simulink model "s5"  (Simulink 2.00)
settings: Solver=ode15s  StartTime=0.0  StopTime=tstop  MaxStep=1e-2  RelTol=1e-6  AbsTol=1e-6
values from neighbouring files (symbols this model uses):
  Domega = 0    [I3ESSR.M]    (also in M3.M; M3G.M; M5.M = 1; SET1.M = 2)
  H = 2.89    [I3ESSR.M]    (also in M1.M = 0.5*J_rotor*wbasem*wbasem/Sbase; M3.M = diag(h); M3G.M = diag(h); M5.M = 0.352825293175)
  IdeIqe = polyfit(Iqe',Ide',2)    [M5.M]
  Ipm = Em/xmd    [M5.M]
  Psido = xls*(-Ido) + Psiado    [M1.M]    (also in M3.M = xls*(-Ido) + Psimdo; M3G.M = xls*(-Ido) + Psimdo; M5.M = Psiado)
  Psiqo = xls*(-Iqo) + Psiaqo    [M1.M]    (also in M3.M = xls*(-Iqo) + Psimqo; M3G.M = xls*(-Iqo) + Psimqo; M5.M = 0)
  rs = 0.00    (= 0)    [I3ESSR.M]    (also in M1.M = rs/Zbase; M3.M; M3G.M = 0.001; M5.M = rs/Zb)
  VsTem = polyfit(Tem',Vs',2)    [M5.M]
  wb = wbase    [M1.M]    (also in M2.M = 376.991118431; M3.M = 376.991118431; M3G.M = 376.991118431; M4.M = we)
  wrbywbo = 0    [M5.M]
  xd = 1.79    [I3ESSR.M]    (also in M1.M = xd/Zbase; M3.M; M3G.M; M5.M = xd/Zb)
  xls = 0.13    [I3ESSR.M]    (also in M1.M = xls/Zbase; M3.M; M3G.M; M5.M = xls/Zb)
  xmd = xmd/Zbase    [M1.M]    (also in M3.M = 1.66; M3G.M = 1.66; M5.M = xmd/Zb)
  xMD = (1/xls + 1/xmd + 1/xplf + 1/xplkd)^(-1)    [M1.M]    (also in M3.M = 0.00484867453082; M3G.M = 0.00484867453082; M5.M = 0.0152325462012)
  xMQ = (1/xls + 1/xmq + 1/xplkq)^(-1)    [M1.M]    (also in M3.M = 0.0456224786115; M3G.M = 0.0456224786115; M5.M = 0.0170549070248)
  xq = 1.71    [I3ESSR.M]    (also in M1.M = xq/Zbase; M3.M; M3G.M; M5.M = xq/Zb)
  Zb = Vb/Ib    [M5.M]
settings Model: SaveTime=off  SaveOutput=off  ConsistencyChecking=off

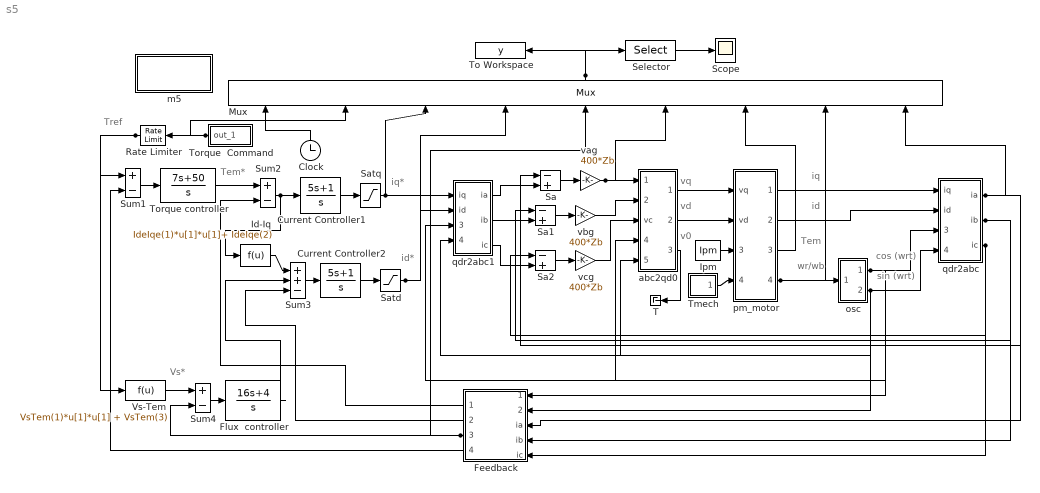
== system s5 ==
  note: Tem
  note: wr/wb
  note: cos (wrt)
  note: sin (wrt)
  note: id
  note: iq
  note: Vs*
  note: Tem*
  note: Tref
  note: id*
  note: iq*
  note: vq
  note: vd
  note: v0
  Clock : Clock
      settings: Orientation=up  DeleteFcn=simclock BlockIsBeingDestroyed  PostSaveFcn=simclock Save
  Current Controller1 : TransferFcn  Numerator=[5 1]  Denominator=[1 0]
  Current Controller2 : TransferFcn  Numerator=[5 1]  Denominator=[1 0]
  Feedback : Subsystem  Orientation=left
  Flux  controller : TransferFcn  Numerator=[16 4]  Denominator=[1 0]
  Id-Iq : Fcn  Expr=IdeIqe(1)*u[1]*u[1]+ IdeIqe(2)
  Ipm : Constant  Value=Ipm
  m5 : Subsystem
      settings: OpenFcn=m5
      mask Type: Masked block of m5.m
      mask Help: Uses m5.m to initialize and plot
      mask Display: disp('Initialize\nand plot')
  Mux : Mux  Orientation=up  Inputs=9
  Rate Limiter : RateLimiter  Orientation=left  RisingSlewLimit=1000  FallingSlewLimit=-1000
  Sa : Sum  Inputs=-+
  Sa1 : Sum  Inputs=-+
  Sa2 : Sum  Inputs=-+
  Satd : Saturate  UpperLimit=1.2  LowerLimit=-1.2
  Satq : Saturate  UpperLimit=1.2  LowerLimit=-1.2
  Scope : Scope
      settings: TickLabels=on  TimeRange=3  YMin=-1  YMax=1  SaveToWorkspace=off  SaveName=ScopeData  LimitMaxRows=off
  Selector : Selector  Elements=[2 5 6 7 8 9]  InputPortWidth=9
  Sum1 : Sum  Inputs=+-
  Sum2 : Sum  Inputs=+-
  Sum3 : Sum  Inputs=++-
  Sum4 : Sum  Inputs=+-
  T : Terminator
  Tmech : Subsystem  mask(Repeating table){@1=tmech_time, @2=tmech_value}
      mask prompts: @1 "Time values:"; @2 "Output values:"
      mask help:
      | Repeating table.
      | Enter values of time and output for first cycle.
      mask init:
      | period = max(@1); t = @1; y = @2;
      mask Help: Repeats cycle given in table. Time values should be monotonically increasing.
      mask Display: plot([t,t+period,t+2*period],[y,y,y])
  To Workspace : ToWorkspace  VariableName=y  SampleTime=0
      settings: Buffer=40000
  Torque controller : TransferFcn  Numerator=[7 50]  Denominator=[1 0]
  Torque  Command : Subsystem  Orientation=left  mask(Repeating table){@1=tref_time, @2=tref_value}
      mask prompts: @1 "Time values:"; @2 "Output values:"
      mask help:
      | Repeating table.
      | Enter values of time and output for first cycle.
      mask init:
      | period = max(@1); t = @1; y = @2;
      mask Help: Repeats cycle given in table. Time values should be monotonically increasing.
      mask Display: plot([t,t+period,t+2*period],[y,y,y])
  Vs-Tem : Fcn  Expr=VsTem(1)*u[1]*u[1] + VsTem(3)
  abc2qd0 : Subsystem
  osc : Subsystem
  pm_motor : Subsystem
  qdr2abc : Subsystem
  qdr2abc1 : Subsystem
  vag : Gain  Gain=400*Zb
  vbg : Gain  Gain=400*Zb
  vcg : Gain  Gain=400*Zb
  wires:
  Mux/1 -> Selector/1, To Workspace/1
  Selector/1 -> Scope/1
  abc2qd0/3(vd0) -> T/1
  pm_motor/4(wr/wb) -> Mux/8, osc/1(wr/wb)
  pm_motor/3(Tem) -> Mux/7
  pm_motor/2(id_motor) -> qdr2abc/2(id)
  Rate Limiter/1 -> Sum1/1, Vs-Tem/1
  Torque  Command/1(out_1) -> Rate Limiter/1, Mux/2
  Satd/1 -> Mux/4, qdr2abc1/2(id)
  Current Controller2/1 -> Satd/1
  Satq/1 -> Mux/3, qdr2abc1/1(iq)
  Current Controller1/1 -> Satq/1
  Feedback/3(out_psigap) -> Mux/5, Sum4/2
  vag/1 -> Mux/6, abc2qd0/1(va)
  Feedback/1(out_iq) -> Sum2/2
  Feedback/2(out_id) -> Sum3/3
  Feedback/4(out_Tem) -> Sum1/2
  Sum2/1 -> Id-Iq/1, Current Controller1/1
  Torque controller/1 -> Sum2/1
  vcg/1 -> abc2qd0/3(vc)
  vbg/1 -> abc2qd0/2(vb)
  osc/1(cos_thetar) -> abc2qd0/4(cos_thetar), qdr2abc1/3(cos(thetar)), Feedback/1(cos_thetar), qdr2abc/3(cos_thetar)
  osc/2(sin_thetar) -> qdr2abc1/4(sin(thetar)), qdr2abc/4(sin_thetar), Feedback/2(sin_thetar), abc2qd0/5(sin_thetar)
  Id-Iq/1 -> Sum3/1
  Flux  controller/1 -> Sum3/2
  Vs-Tem/1 -> Sum4/1
  Sum4/1 -> Flux  controller/1
  Sum3/1 -> Current Controller2/1
  qdr2abc/3(ic) -> Feedback/5(ic), Sa2/1
  qdr2abc/2(ib) -> Feedback/4(ib), Sa1/1
  qdr2abc/1(ia) -> Mux/9, Feedback/3(ia), Sa/1
  qdr2abc1/3(ic) -> Sa2/2
  qdr2abc1/2(ib) -> Sa1/2
  Tmech/1(out_1) -> pm_motor/4(Tmech)
  Ipm/1 -> pm_motor/3(Ipm)
  pm_motor/1(iq_motor) -> qdr2abc/1(iq)
  abc2qd0/1(vq) -> pm_motor/1(vq)
  abc2qd0/2(vd) -> pm_motor/2(vd)
  Sum1/1 -> Torque controller/1
  Sa2/1 -> vcg/1
  Sa/1 -> vag/1
  Sa1/1 -> vbg/1
  qdr2abc1/1(ia) -> Sa/2
  Clock/1 -> Mux/1

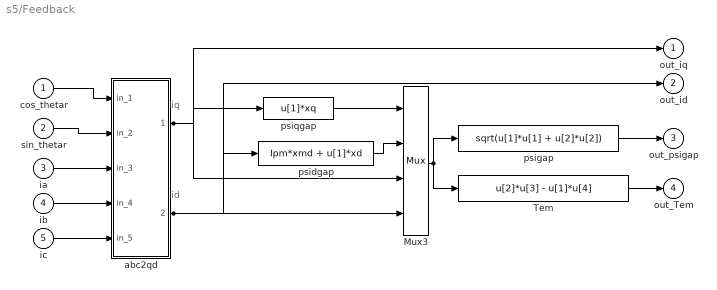
== system s5/Feedback ==
  note: id
  note: iq
  cos_thetar : Inport  Port=1  PortWidth=-1  SampleTime=-1
  sin_thetar : Inport  Port=2  PortWidth=-1  SampleTime=-1
  ia : Inport  Port=3  PortWidth=-1  SampleTime=-1
  ib : Inport  Port=4  PortWidth=-1  SampleTime=-1
  ic : Inport  Port=5  PortWidth=-1  SampleTime=-1
  Mux3 : Mux  Inputs=4
  Tem : Fcn  Expr=u[2]*u[3] - u[1]*u[4]
  abc2qd : Subsystem
  psidgap : Fcn  Expr=Ipm*xmd + u[1]*xd
  psigap : Fcn  Expr=sqrt(u[1]*u[1] + u[2]*u[2])
  psiqgap : Fcn  Expr=u[1]*xq
  out_iq : Outport  Port=1  InitialOutput=0
  out_id : Outport  Port=2  InitialOutput=0
  out_psigap : Outport  Port=3  InitialOutput=0
  out_Tem : Outport  Port=4  InitialOutput=0
  wires:
  abc2qd/2(out_id) -> psidgap/1, out_id/1, Mux3/4
  abc2qd/1(out_iq) -> psiqgap/1, out_iq/1, Mux3/3
  psigap/1 -> out_psigap/1
  Tem/1 -> out_Tem/1
  Mux3/1 -> psigap/1, Tem/1
  psidgap/1 -> Mux3/2
  psiqgap/1 -> Mux3/1
  sin_thetar/1 -> abc2qd/2(in_2)
  cos_thetar/1 -> abc2qd/1(in_1)
  ic/1 -> abc2qd/5(in_5)
  ib/1 -> abc2qd/4(in_4)
  ia/1 -> abc2qd/3(in_3)

== system s5/m5 ==
  note: Masked block m5.m to initialize
      | s5.m in Chapter 10 and to plot results

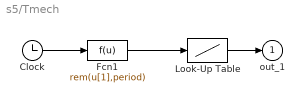
== system s5/Tmech ==
  Clock : Clock
      settings: DeleteFcn=simclock BlockIsBeingDestroyed  PostSaveFcn=simclock Save
  Fcn1 : Fcn  Expr=rem(u[1],period)
  Look-Up Table : Lookup  InputValues=t  OutputValues=y
  out_1 : Outport  Port=1  InitialOutput=0
  wires:
  Fcn1/1 -> Look-Up Table/1
  Clock/1 -> Fcn1/1
  Look-Up Table/1 -> out_1/1

== system s5/Torque  Command ==
  Clock : Clock
      settings: DeleteFcn=simclock BlockIsBeingDestroyed  PostSaveFcn=simclock Save
  Fcn1 : Fcn  Expr=rem(u[1],period)
  Look-Up Table : Lookup  InputValues=t  OutputValues=y
  out_1 : Outport  Port=1  InitialOutput=0
  wires:
  Fcn1/1 -> Look-Up Table/1
  Clock/1 -> Fcn1/1
  Look-Up Table/1 -> out_1/1

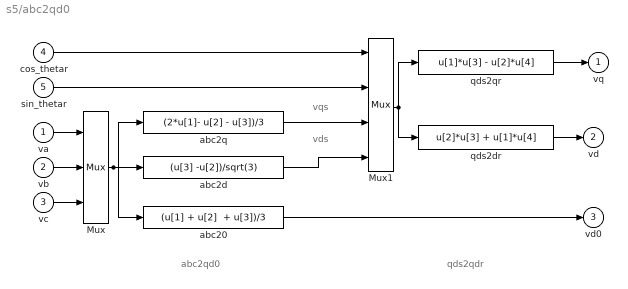
== system s5/abc2qd0 ==
  note: vqs
  note: qds2qdr
  note: abc2qd0
  note: vds
  va : Inport  Port=1  PortWidth=-1  SampleTime=-1
  vb : Inport  Port=2  PortWidth=-1  SampleTime=-1
  vc : Inport  Port=3  PortWidth=-1  SampleTime=-1
  cos_thetar : Inport  Port=4  PortWidth=-1  SampleTime=-1
  sin_thetar : Inport  Port=5  PortWidth=-1  SampleTime=-1
  Mux : Mux  Inputs=3
  Mux1 : Mux  Inputs=4
  abc20 : Fcn  Expr="(u[1] + u[2]  + u[3])/3"
  abc2d : Fcn  Expr=(u[3] -u[2])/sqrt(3)
  abc2q : Fcn  Expr=(2*u[1]- u[2] - u[3])/3
  qds2dr : Fcn  Expr=u[2]*u[3] + u[1]*u[4]
  qds2qr : Fcn  Expr=u[1]*u[3] - u[2]*u[4]
  vq : Outport  Port=1  InitialOutput=0
  vd : Outport  Port=2  InitialOutput=0
  vd0 : Outport  Port=3  InitialOutput=0
  wires:
  abc20/1 -> vd0/1
  abc2d/1 -> Mux1/4
  abc2q/1 -> Mux1/3
  sin_thetar/1 -> Mux1/2
  cos_thetar/1 -> Mux1/1
  qds2dr/1 -> vd/1
  qds2qr/1 -> vq/1
  vc/1 -> Mux/3
  vb/1 -> Mux/2
  va/1 -> Mux/1
  Mux1/1 -> qds2dr/1, qds2qr/1
  Mux/1 -> abc20/1, abc2d/1, abc2q/1

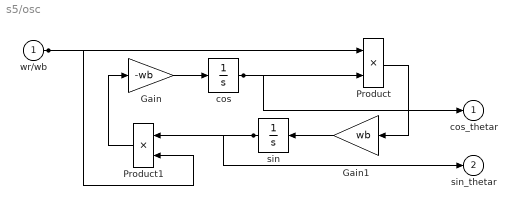
== system s5/osc ==
  wr/wb : Inport  Port=1  PortWidth=-1  SampleTime=-1
  Gain : Gain  Gain=-wb
  Gain1 : Gain  Orientation=left  Gain=wb
  Product : Product  Inputs=2
  Product1 : Product  Orientation=left  Inputs=2
  cos : Integrator  ExternalReset=none  InitialConditionSource=internal  InitialCondition=1  LimitOutput=off  UpperSaturationLimit=inf  LowerSaturationLimit=-inf  ShowSaturationPort=off  ShowStatePort=off  AbsoluteTolerance=auto
  sin : Integrator  Orientation=left  ExternalReset=none  InitialConditionSource=internal  InitialCondition=0  LimitOutput=off  UpperSaturationLimit=inf  LowerSaturationLimit=-inf  ShowSaturationPort=off  ShowStatePort=off  AbsoluteTolerance=auto
  cos_thetar : Outport  Port=1  InitialOutput=0
  sin_thetar : Outport  Port=2  InitialOutput=0
  wires:
  sin/1 -> sin_thetar/1, Product1/1
  wr/wb/1 -> Product1/2, Product/1
  Gain1/1 -> sin/1
  Product1/1 -> Gain/1
  Gain/1 -> cos/1
  cos/1 -> Product/2, cos_thetar/1
  Product/1 -> Gain1/1

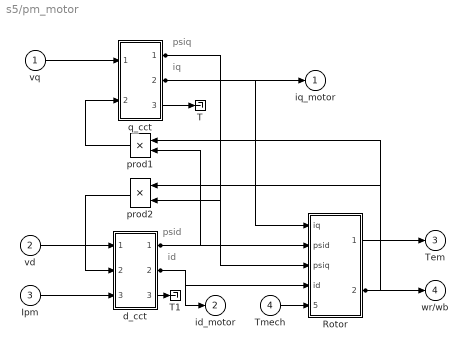
== system s5/pm_motor ==
  note: psiq
  note: iq
  note: id
  note: psid
  vq : Inport  Port=1  PortWidth=-1  SampleTime=-1
  vd : Inport  Port=2  PortWidth=-1  SampleTime=-1
  Ipm : Inport  Port=3  PortWidth=-1  SampleTime=-1
  Tmech : Inport  Port=4  PortWidth=-1  SampleTime=-1
  Rotor : Subsystem
  T : Terminator
  T1 : Terminator
  d_cct : Subsystem
  prod1 : Product  Orientation=left  Inputs=2
  prod2 : Product  Orientation=left  Inputs=2
  q_cct : Subsystem
  iq_motor : Outport  Port=1  InitialOutput=0
  id_motor : Outport  Port=2  InitialOutput=0
  Tem : Outport  Port=3  InitialOutput=0
  wr/wb : Outport  Port=4  InitialOutput=0
  wires:
  d_cct/3(Out_psimd) -> T1/1
  q_cct/3(Out_psimq) -> T/1
  Rotor/1(Tem) -> Tem/1
  Rotor/2("wr/wb ") -> wr/wb/1, prod2/1, prod1/1
  prod2/1 -> d_cct/2(In_wrpsiq)
  vd/1 -> d_cct/1(In_vd)
  Ipm/1 -> d_cct/3(In_Ipm)
  q_cct/1(Out_psiq) -> prod2/2, Rotor/3(psiq)
  d_cct/1(Out_psid) -> prod1/2, Rotor/2("psid ")
  vq/1 -> q_cct/1(In_vq)
  prod1/1 -> q_cct/2(In_wrpsid)
  d_cct/2(Out_id) -> id_motor/1, Rotor/4(id)
  q_cct/2(Out_iq) -> iq_motor/1, Rotor/1(iq)
  Tmech/1 -> Rotor/5(Tmech)

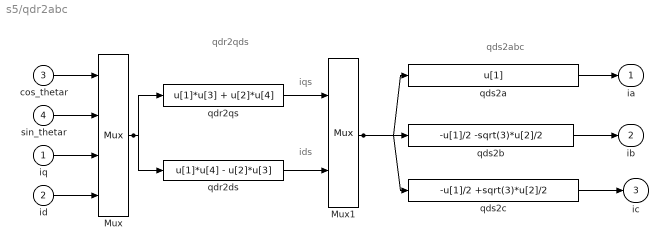
== system s5/qdr2abc ==
  note: ids
  note: iqs
  note: qds2abc
  note: qdr2qds
  iq : Inport  Port=1  PortWidth=-1  SampleTime=-1
  id : Inport  Port=2  PortWidth=-1  SampleTime=-1
  cos_thetar : Inport  Port=3  PortWidth=-1  SampleTime=-1
  sin_thetar : Inport  Port=4  PortWidth=-1  SampleTime=-1
  Mux : Mux  Inputs=4
  Mux1 : Mux  Inputs=2
  qdr2ds : Fcn  Expr=u[1]*u[4] - u[2]*u[3]
  qdr2qs : Fcn  Expr=u[1]*u[3] + u[2]*u[4]
  qds2a : Fcn  Expr=u[1]
  qds2b : Fcn  Expr=-u[1]/2 -sqrt(3)*u[2]/2
  qds2c : Fcn  Expr=-u[1]/2 +sqrt(3)*u[2]/2
  ia : Outport  Port=1  InitialOutput=0
  ib : Outport  Port=2  InitialOutput=0
  ic : Outport  Port=3  InitialOutput=0
  wires:
  qds2c/1 -> ic/1
  qds2b/1 -> ib/1
  qds2a/1 -> ia/1
  Mux1/1 -> qds2c/1, qds2a/1, qds2b/1
  qdr2ds/1 -> Mux1/2
  qdr2qs/1 -> Mux1/1
  Mux/1 -> qdr2ds/1, qdr2qs/1
  id/1 -> Mux/4
  iq/1 -> Mux/3
  sin_thetar/1 -> Mux/2
  cos_thetar/1 -> Mux/1

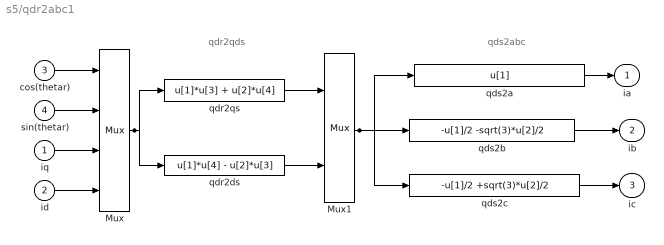
== system s5/qdr2abc1 ==
  note: qdr2qds
  note: qds2abc
  iq : Inport  Port=1  PortWidth=-1  SampleTime=-1
  id : Inport  Port=2  PortWidth=-1  SampleTime=-1
  cos(thetar) : Inport  Port=3  PortWidth=-1  SampleTime=-1
  sin(thetar) : Inport  Port=4  PortWidth=-1  SampleTime=-1
  Mux : Mux  Inputs=4
  Mux1 : Mux  Inputs=2
  qdr2ds : Fcn  Expr=u[1]*u[4] - u[2]*u[3]
  qdr2qs : Fcn  Expr=u[1]*u[3] + u[2]*u[4]
  qds2a : Fcn  Expr=u[1]
  qds2b : Fcn  Expr=-u[1]/2 -sqrt(3)*u[2]/2
  qds2c : Fcn  Expr=-u[1]/2 +sqrt(3)*u[2]/2
  ia : Outport  Port=1  InitialOutput=0
  ib : Outport  Port=2  InitialOutput=0
  ic : Outport  Port=3  InitialOutput=0
  wires:
  qds2c/1 -> ic/1
  qds2b/1 -> ib/1
  qds2a/1 -> ia/1
  Mux1/1 -> qds2c/1, qds2a/1, qds2b/1
  qdr2ds/1 -> Mux1/2
  qdr2qs/1 -> Mux1/1
  Mux/1 -> qdr2ds/1, qdr2qs/1
  id/1 -> Mux/4
  iq/1 -> Mux/3
  sin(thetar)/1 -> Mux/2
  cos(thetar)/1 -> Mux/1

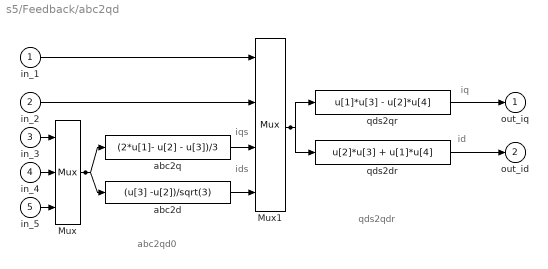
== system s5/Feedback/abc2qd ==
  note: iq
  note: id
  note: ids
  note: iqs
  note: qds2qdr
  note: abc2qd0
  in_1 : Inport  Port=1  PortWidth=-1  SampleTime=-1
  in_2 : Inport  Port=2  PortWidth=-1  SampleTime=-1
  in_3 : Inport  Port=3  PortWidth=-1  SampleTime=-1
  in_4 : Inport  Port=4  PortWidth=-1  SampleTime=-1
  in_5 : Inport  Port=5  PortWidth=-1  SampleTime=-1
  Mux : Mux  Inputs=3
  Mux1 : Mux  Inputs=4
  abc2d : Fcn  Expr=(u[3] -u[2])/sqrt(3)
  abc2q : Fcn  Expr=(2*u[1]- u[2] - u[3])/3
  qds2dr : Fcn  Expr=u[2]*u[3] + u[1]*u[4]
  qds2qr : Fcn  Expr=u[1]*u[3] - u[2]*u[4]
  out_iq : Outport  Port=1  InitialOutput=0
  out_id : Outport  Port=2  InitialOutput=0
  wires:
  in_5/1 -> Mux/3
  in_4/1 -> Mux/2
  qds2dr/1 -> out_id/1
  in_3/1 -> Mux/1
  in_2/1 -> Mux1/2
  qds2qr/1 -> out_iq/1
  in_1/1 -> Mux1/1
  Mux/1 -> abc2q/1, abc2d/1
  Mux1/1 -> qds2qr/1, qds2dr/1
  abc2q/1 -> Mux1/3
  abc2d/1 -> Mux1/4

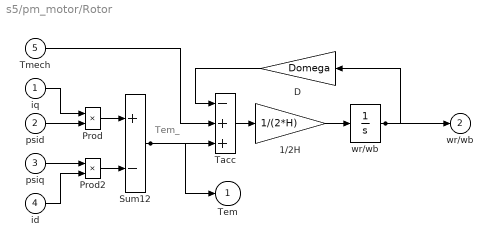
== system s5/pm_motor/Rotor ==
  note: Tem_
  iq : Inport  Port=1  PortWidth=-1  SampleTime=-1
  "psid " : Inport  Port=2  PortWidth=-1  SampleTime=-1
  psiq : Inport  Port=3  PortWidth=-1  SampleTime=-1
  id : Inport  Port=4  PortWidth=-1  SampleTime=-1
  Tmech : Inport  Port=5  PortWidth=-1  SampleTime=-1
  1/2H : Gain  Gain=1/(2*H)
  D : Gain  Orientation=left  Gain=Domega
  Prod : Product  Inputs=2
  Prod2 : Product  Inputs=2
  Sum12 : Sum  Inputs=+-
  Tacc : Sum  Inputs=-++
  wr/wb : Integrator  ExternalReset=none  InitialConditionSource=internal  InitialCondition=wrbywbo  LimitOutput=off  UpperSaturationLimit=inf  LowerSaturationLimit=-inf  ShowSaturationPort=off  ShowStatePort=off  AbsoluteTolerance=auto
  Tem : Outport  Port=1  InitialOutput=0
  "wr/wb " : Outport  Port=2  InitialOutput=0
  wires:
  wr/wb/1 -> "wr/wb "/1, D/1
  Tmech/1 -> Tacc/2
  Sum12/1 -> Tem/1, Tacc/3
  id/1 -> Prod2/2
  psiq/1 -> Prod2/1
  "psid "/1 -> Prod/2
  iq/1 -> Prod/1
  Prod/1 -> Sum12/1
  Tacc/1 -> 1/2H/1
  1/2H/1 -> wr/wb/1
  Prod2/1 -> Sum12/2
  D/1 -> Tacc/1

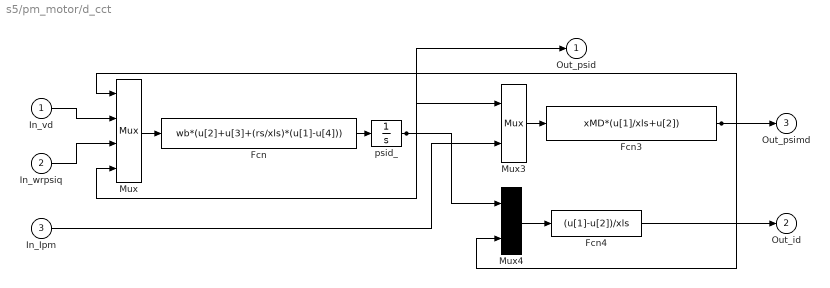
== system s5/pm_motor/d_cct ==
  In_vd : Inport  Port=1  PortWidth=-1  SampleTime=-1
  In_wrpsiq : Inport  Port=2  PortWidth=-1  SampleTime=-1
  In_Ipm : Inport  Port=3  PortWidth=-1  SampleTime=-1
  Fcn : Fcn  Expr=wb*(u[2]+u[3]+(rs/xls)*(u[1]-u[4]))
  Fcn3 : Fcn  Expr=xMD*(u[1]/xls+u[2])
  Fcn4 : Fcn  Expr=(u[1]-u[2])/xls
  Mux : Mux  Inputs=4
  Mux3 : Mux  Inputs=2
  Mux4 : Mux  Inputs=2
  psid_ : Integrator  ExternalReset=none  InitialConditionSource=internal  InitialCondition=Psido  LimitOutput=off  UpperSaturationLimit=inf  LowerSaturationLimit=-inf  ShowSaturationPort=off  ShowStatePort=off  AbsoluteTolerance=auto
  Out_psid : Outport  Port=1  InitialOutput=0
  Out_id : Outport  Port=2  InitialOutput=0
  Out_psimd : Outport  Port=3  InitialOutput=0
  wires:
  In_Ipm/1 -> Mux3/2
  Fcn4/1 -> Out_id/1
  Fcn3/1 -> Out_psimd/1, Mux/1, Mux4/2
  Mux4/1 -> Fcn4/1
  Mux3/1 -> Fcn3/1
  psid_/1 -> Out_psid/1, Mux4/1, Mux3/1, Mux/4
  Fcn/1 -> psid_/1
  Mux/1 -> Fcn/1
  In_vd/1 -> Mux/2
  In_wrpsiq/1 -> Mux/3

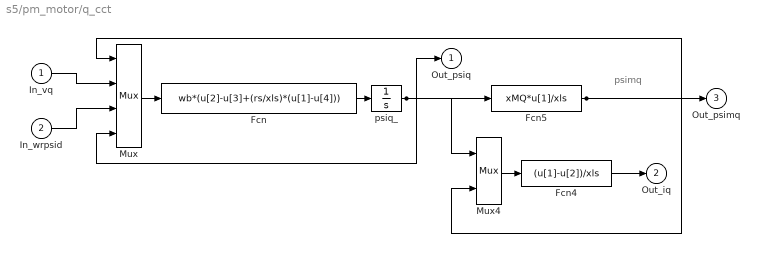
== system s5/pm_motor/q_cct ==
  note: psimq
  In_vq : Inport  Port=1  PortWidth=-1  SampleTime=-1
  In_wrpsid : Inport  Port=2  PortWidth=-1  SampleTime=-1
  Fcn : Fcn  Expr=wb*(u[2]-u[3]+(rs/xls)*(u[1]-u[4]))
  Fcn4 : Fcn  Expr=(u[1]-u[2])/xls
  Fcn5 : Fcn  Expr=xMQ*u[1]/xls
  Mux : Mux  Inputs=4
  Mux4 : Mux  Inputs=2
  psiq_ : Integrator  ExternalReset=none  InitialConditionSource=internal  InitialCondition=Psiqo  LimitOutput=off  UpperSaturationLimit=inf  LowerSaturationLimit=-inf  ShowSaturationPort=off  ShowStatePort=off  AbsoluteTolerance=auto
  Out_psiq : Outport  Port=1  InitialOutput=0
  Out_iq : Outport  Port=2  InitialOutput=0
  Out_psimq : Outport  Port=3  InitialOutput=0
  wires:
  Fcn5/1 -> Out_psimq/1, Mux/1, Mux4/2
  Fcn4/1 -> Out_iq/1
  psiq_/1 -> Fcn5/1, Out_psiq/1, Mux4/1, Mux/4
  Mux4/1 -> Fcn4/1
  Fcn/1 -> psiq_/1
  Mux/1 -> Fcn/1
  In_vq/1 -> Mux/2
  In_wrpsid/1 -> Mux/3
